simulink library "SingleDotFinder_ul"  (R2018b)
settings: Solver=VariableStepAuto  StartTime=0.0  StopTime=10.0  RelTol=1e-3
undefined symbols (not defined in the file or in its folder): Ignore, masks, vision
libraries: $bdroot x3, simulink x2
settings Model: Creator=mcobb  LastModifiedBy=Owner
settings DebuggingCC: LibraryContextMissingDiagnostic=none
settings SFSimCC: SimUseLocalCustomCode=off
settings RTWCC: RTWUseLocalCustomCode=off

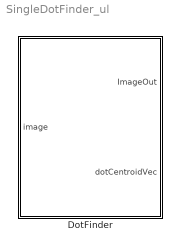
== system SingleDotFinder_ul ==
  DotFinder : Subsystem  mask{ROIPositionHoldEnable=on, ROIPositionHoldCoordinates=[500 500], ROIDimVec_px=[30 90], ROIHalfDimVec_px=[15 45], ROISplitDims_px=[1 15 ; 1 90 ; 16 14 ; 1 90], DotOrientation=Vertical, OverlayOutput=on, ImageDimensions=[765 998], CrosshairPixelWidth_px=1}
      mask prompts: ROIPositionHoldEnable "Hold Position Enable"; ROIPositionHoldCoordinates "Hold Position Coordinates  [rows cols]  (pixels)"; ROIDimVec_px "Dimensions [rows cols]  (pixels)"; ROIHalfDimVec_px "Half Dims  [rows cols]  (pixels)"; ROISplitDims_px "Split Dims [rows cols]  (pixels)"; DotOrientation "Dot Orientation"; OverlayOutput "Draw Output Overlay"; ImageDimensions "Image Dimensions [rows cols] pixels"; CrosshairPixelWidth_px "Crosshair Width (pixels)"
      mask init:
      | dotFinder_init
      mask TypeOptions DotOrientation: Horizontal | Vertical
      mask DialogControl ParameterGroupVar Prompt: Region Of Interest (ROI) Parameters
      mask DialogControl Container3 Prompt: Other Parameters

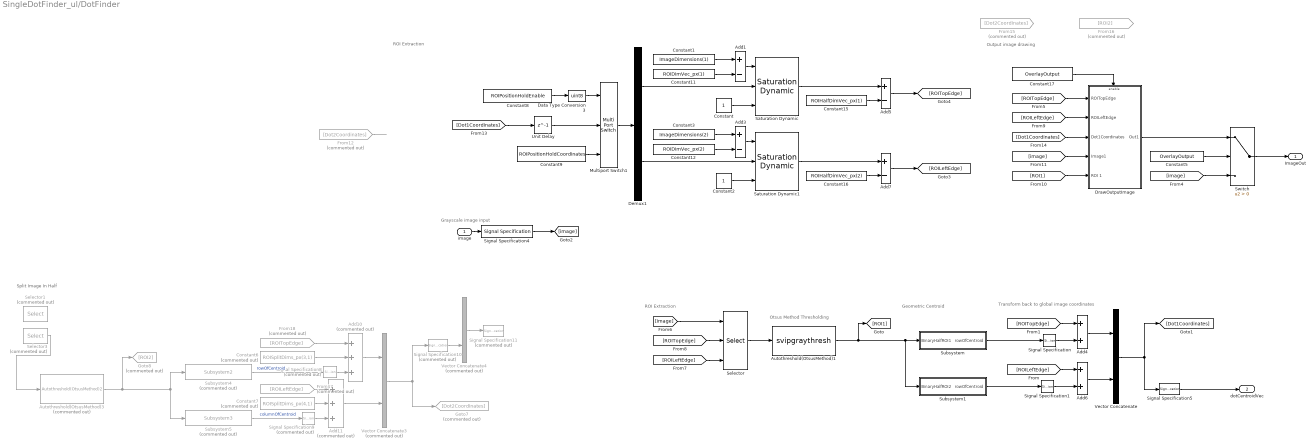
== system SingleDotFinder_ul/DotFinder ==
  note: Transform back to global image coordinates
  note: Geometric Centroid
  note: Otsus Method Thresholding
  note: Split Image
      | In Half
  note: ROI Extraction
  note: Output image drawing
  note: ROI Extraction
  note: Grayscale image input
  image : Inport
  Add{1,3,5,7} (4 alike) : Sum  Inputs=+-
  Add10 : Sum  Commented=on  Inputs=+++
  Add11 : Sum  Commented=on  Inputs=+++
  Add4 : Sum
  Add6 : Sum
  Autothreshold(OtsusMethod)1 : S-Function  DialogController=vipDDGCreate  FunctionName=svipgraythresh  Parameters=operator, userDefinedRange, umin, umax, threshOut, effMetricOut, outOfRngOpt, scaleThreshold, scaleFactor, P1Mode, P1WordLength, P1FracLength, A1Mode, A1WordLength, A1FracLength, P2Mode, P2WordLength, P2FracLength, A2Mode, A2WordLength, A2FracLength, P3Mode, P3WordLength, P3FracLength, A3Mode, A3WordLength, A3FracLength, P4Mode, P4WordLength, P4FracLength, A4Mode, A4WordLength, A4FracLength, Q1Mode, Q1WordLength, Q1FracLength, EMMode, EMWordLength, EMFracLength, dtInfo.roundingMode, dtInfo.overflowMode  SFunctionDeploymentMode=off  EnableBusSupport=off  mask(Autothreshold){operator=>, threshOut=off, effMetricOut=off, userDefinedRange=off, umin=0, umax=255, outOfRngOpt=vision:masks:Ignore, scaleThreshold=off, scaleFactor=1, P1Mode=Specify word length, P1WordLength=32, P1FracLength=30, A1Mode=Same as Product 1, A1WordLength=32, A1FracLength=30, P2Mode=Specify word length, P2WordLength=32, P2FracLength=22, A2Mode=Same as Product 2, A2WordLength=32, A2FracLength=22, P3Mode=Specify word length, P3WordLength=32, P3FracLength=14, A3Mode=Same as Product 3, A3WordLength=32, A3FracLength=14, P4Mode=Binary point scaling, P4WordLength=32, P4FracLength=15, A4Mode=Same as Product 4, A4WordLength=16, A4FracLength=4, Q1Mode=Specify word length, Q1WordLength=32, Q1FracLength=16, EMMode=Specify word length, EMWordLength=16, EMFracLength=14, roundingMode=Floor, overflowMode=off, LockScale=off}
      mask prompts: operator "vision:masks:ThresholdingOperator"; threshOut "vision:masks:OutputThreshold"; effMetricOut "vision:masks:OutputEffectivenessMetric"; userDefinedRange "vision:masks:SpecifyDataRange"; umin "vision:masks:MinimumValueOfInput"; umax "vision:masks:MinimumValueOfInput"; outOfRngOpt "vision:masks:WhenDataRangeIsExceeded"; scaleThreshold "vision:masks:ScaleThreshold_MP"; scaleFactor "vision:masks:ThresholdScalingFactor"; P1Mode "P1:"; P1WordLength "P1 WL:"; P1FracLength "P1 FL:"; A1Mode "A1:"; A1WordLength "A1 WL:"; A1FracLength "A1 FL:"; P2Mode "P2:"; P2WordLength "P2 WL:"; P2FracLength "P2 FL:"; A2Mode "A2:"; A2WordLength "A2 WL:"; A2FracLength "A2 FL:"; P3Mode "P3:"; P3WordLength "P3 WL:"; P3FracLength "P3 FL:"; A3Mode "A3:"; A3WordLength "A3 WL:"; A3FracLength "A3 FL:"; P4Mode "P4:"; P4WordLength "P4 WL:"; P4FracLength "P4 FL:"; A4Mode "A4:"; A4WordLength "A4 WL:"; A4FracLength "A4 FL:"; Q1Mode "Q1:"; Q1WordLength "Q1 WL:"; Q1FracLength "Q1 FL:"; EMMode "EM:"; EMWordLength "EM WL:"; EMFracLength "EM FL:"; roundingMode "vision:masks:RoundIntegerCalculationsTowards"; overflowMode "vision:masks:RoundIntegerCalculationsTowards"; LockScale "vision:masks:LockScaling"
      mask help: vision:masks:AutoThresholdDescription
      mask init:
      | blk = gcbh;
      | 
      | dtInfo = dspGetFixptDataTypeInfo(blk,1);
      | 
      | effMetricOut_str = get_param(blk,'effMetricOut');
      | threshOut_str = get_param(blk,'threshOut');
      | if strcmp(effMetricOut_str,'off') && strcmp(threshOut_str,'off')
      | 	[so(1:3).port] = deal(1,1,1);
      | 	[so(1:3).txt] = deal('BW','BW','BW');
      | elseif strcmp(effMetricOut_str,'on') && strcmp(threshOut_str,'off')
      | 	[so(1:3).port] = deal(1,2,2);
      | 	[so(1:3).txt] = deal('BW','EMetric','EMetric');
      | elseif strcmp(effMetricOut_str,'off') && strcmp(threshOut_str,'on')
      | 	[so(1:3).port] = deal(1,2,2);
      | 	[so(1:3).txt] = deal('BW','Th','Th');
      | else
      | 	[so(1:3).port] = deal(1,2,3);
      | 	[so(1:3).txt] = deal('BW','Th','EMetric');
      | end
      mask Help: eval('visionblockhelp');
      mask TypeOptions operator: > | <=
      mask TypeOptions outOfRngOpt: vision:masks:Ignore | vision:masks:Saturate | vision:masks:WarnAndSaturate | vision:masks:Error
      mask TypeOptions P1Mode: Specify word length | Binary point scaling | Slope and bias scaling
      mask TypeOptions A1Mode: Same as Product 1 | Specify word length | Binary point scaling | Slope and bias scaling
      mask TypeOptions P2Mode: Specify word length | Binary point scaling | Slope and bias scaling
      mask TypeOptions A2Mode: Same as Product 2 | Specify word length | Binary point scaling | Slope and bias scaling
      mask TypeOptions P3Mode: Specify word length | Binary point scaling | Slope and bias scaling
      mask TypeOptions A3Mode: Same as Product 3 | Specify word length | Binary point scaling | Slope and bias scaling
      mask TypeOptions P4Mode: Same as input | Binary point scaling | Slope and bias scaling
      mask TypeOptions A4Mode: Same as Product 4 | Binary point scaling | Slope and bias scaling
      mask TypeOptions Q1Mode: Specify word length | Binary point scaling | Slope and bias scaling
      mask TypeOptions EMMode: Specify word length | Binary point scaling | Slope and bias scaling
      mask TypeOptions roundingMode: dspshared:FixptDialog:Ceiling_CB | dspshared:FixptDialog:Convergent_CB | dspshared:FixptDialog:Floor_CB | dspshared:FixptDialog:Nearest_CB | dspshared:FixptDialog:Round_CB | dspshared:FixptDialog:Simplest_CB | dspshared:FixptDialog:Zero_CB
      mask Display:
      | disp('Autothreshold');
      | port_label('input',1,'I');
      | port_label('output',so(1).port, so(1).txt);
      | port_label('output',so(2).port, so(2).txt);
      | port_label('output',so(3).port, so(3).txt);
  Autothreshold(OtsusMethod)3 : $bdroot/DotFinder/Autothreshold(OtsusMethod)2  Commented=on  operator=>  threshOut=off  effMetricOut=off  userDefinedRange=off  umin=0  umax=255  outOfRngOpt=vision:masks:Ignore  scaleThreshold=off  scaleFactor=1  P1Mode=Specify word length  P1WordLength=32  P1FracLength=30  P2Mode=Specify word length  P2WordLength=32  P2FracLength=22  P3Mode=Specify word length  P3WordLength=32  P3FracLength=14  P4Mode=Binary point scaling  P4WordLength=32  P4FracLength=15  Q1Mode=Specify word length  Q1WordLength=32  Q1FracLength=16  EMMode=Specify word length  EMWordLength=16  EMFracLength=14  roundingMode=Floor  overflowMode=off
  Constant : Constant
  Constant1 : Constant  Value=ImageDimensions(1)
  Constant11 : Constant  Value=ROIDimVec_px(1)
  Constant12 : Constant  Value=ROIDimVec_px(2)
  Constant15 : Constant  Value=ROIHalfDimVec_px(1)
  Constant16 : Constant  Value=ROIHalfDimVec_px(2)
  Constant17 : Constant  Value=OverlayOutput
  Constant2 : Constant
  Constant3 : Constant  Value=ImageDimensions(2)
  Constant5 : Constant  Value=OverlayOutput
  Constant6 : Constant  Commented=on  Value=ROISplitDims_px(3,1)
  Constant7 : Constant  Commented=on  Value=ROISplitDims_px(4,1)
  Constant8 : Constant  Value=ROIPositionHoldEnable
  Constant9 : Constant  Value=ROIPositionHoldCoordinates
  Data Type Conversion3 : DataTypeConversion  OutDataTypeStr=uint8
  Demux1 : Demux  Outputs=2
  DrawOutputImage : Subsystem
  From12 : From  Commented=on  GotoTag=Dot2Coordinates
  From15 : From  Commented=on  GotoTag=Dot2Coordinates
  From16 : From  Commented=on  GotoTag=ROI2
  From17 : From  Commented=on  GotoTag=ROILeftEdge
  From18 : From  Commented=on  GotoTag=ROITopEdge
  Goto7 : Goto  Commented=on  GotoTag=Dot2Coordinates
  Goto8 : Goto  Commented=on  GotoTag=ROI2
  Multiport Switch1 : MultiPortSwitch  DataPortOrder=Zero-based contiguous  Inputs=2  zeroidx=on
  Saturation Dynamic : simulink/Discontinuities/Saturation Dynamic  OutMin=[]  OutMax=[]  OutDataTypeStr=Inherit: Same as second input  OutDataType=fixdt(1, 16)  OutScaling=2^-10  DoSatur=off
  Saturation Dynamic1 : simulink/Discontinuities/Saturation Dynamic  OutMin=[]  OutMax=[]  OutDataTypeStr=Inherit: Same as second input  OutDataType=fixdt(1, 16)  OutScaling=2^-10  DoSatur=off
  Selector : Selector  NumberOfDimensions=2  InputPortWidth=3  IndexOptions=Starting index (port),Starting index (port)  Indices=[1 3],1  OutputSizes=ROIDimVec_px(1),ROIDimVec_px(2)
  Selector1 : Selector  Commented=on  NumberOfDimensions=2  InputPortWidth=3  IndexOptions=Starting index (dialog),Starting index (dialog)  Indices=ROISplitDims_px(1,1),ROISplitDims_px(2,1)  OutputSizes=ROISplitDims_px(1,2),ROISplitDims_px(2,2)
  Selector3 : Selector  Commented=on  NumberOfDimensions=2  InputPortWidth=3  IndexOptions=Starting index (dialog),Starting index (dialog)  Indices=ROISplitDims_px(3,1),ROISplitDims_px(4,1)  OutputSizes=ROISplitDims_px(3,2),ROISplitDims_px(4,2)
  Signal Specification : SignalSpecification  Dimensions=1
  Signal Specification1 : SignalSpecification  Dimensions=1
  Signal Specification10 : SignalSpecification  Commented=on  Dimensions=[1 2]
  Signal Specification11 : SignalSpecification  Commented=on  Dimensions=[1 4]
  Signal Specification4 : SignalSpecification  Dimensions=ImageDimensions
  Signal Specification5 : SignalSpecification  Dimensions=[1 2]
  Signal Specification8 : SignalSpecification  Commented=on  Dimensions=1
  Signal Specification9 : SignalSpecification  Commented=on  Dimensions=1
  Subsystem : Subsystem
  Subsystem1 : Subsystem
  Subsystem4 : $bdroot/DotFinder/Subsystem2  Commented=on  SystemSampleTime=-1  SSRTWFcnClass=[]
  Subsystem5 : $bdroot/DotFinder/Subsystem3  Commented=on  SystemSampleTime=-1  SSRTWFcnClass=[]
  Switch : Switch  Criteria=u2 > Threshold
  Unit Delay : Delay  DelayLength=1  InitialCondition=ROIPositionHoldCoordinates
  Vector Concatenate : Concatenate
  Vector Concatenate3 : Concatenate  Commented=on
  Vector Concatenate4 : Concatenate  Commented=on  ConcatenateDimension=2
  ImageOut : Outport  PortDimensions=ImageDimensions
  dotCentroidVec : Outport  Port=2
  wires:
  Data Type Conversion3/1 -> Multiport Switch1/1
  Unit Delay/1 -> Multiport Switch1/2
  Multiport Switch1/1 -> Demux1/1
  Demux1/1 -> Saturation Dynamic/2
  Constant/1 -> Saturation Dynamic/3
  Constant1/1 -> Add1/1
  Constant11/1 -> Add1/2
  Constant12/1 -> Add3/2
  Constant3/1 -> Add3/1
  Demux1/2 -> Saturation Dynamic1/2
  Constant15/1 -> Add5/2
  Constant16/1 -> Add7/2
  [image] -> Selector/1
  Constant8/1 -> Data Type Conversion3/1
  Constant9/1 -> Multiport Switch1/3
  Saturation Dynamic/1 -> Add5/1
  Saturation Dynamic1/1 -> Add7/1
  Constant2/1 -> Saturation Dynamic1/3
  Add3/1 -> Saturation Dynamic1/1
  Add1/1 -> Saturation Dynamic/1
  Subsystem1/1(rowOfCentroid) -> Signal Specification1/1
  [ROITopEdge] -> Add4/1
  [ROILeftEdge] -> Add6/1
  Add4/1 -> Vector Concatenate/1
  Add6/1 -> Vector Concatenate/2
  image/1 -> Signal Specification4/1
  Add7/1 -> [ROILeftEdge]
  Add5/1 -> [ROITopEdge]
  Constant17/1 -> DrawOutputImage/Enable
  DrawOutputImage/1(Out1) -> Switch/1
  [ROILeftEdge] -> Selector/3
  [ROITopEdge] -> Selector/2
  [ROITopEdge] -> DrawOutputImage/1(ROITopEdge)
  [ROILeftEdge] -> DrawOutputImage/2(ROILeftEdge)
  [ROI1] -> DrawOutputImage/5("ROI 1 ")
  [image] -> Switch/3
  Constant5/1 -> Switch/2
  [image] -> DrawOutputImage/4(Image1)
  Vector Concatenate/1 -> Signal Specification5/1, [Dot1Coordinates]
  [Dot1Coordinates] -> DrawOutputImage/3(Dot1Coordinates)
  Switch/1 -> ImageOut/1
  Signal Specification/1 -> Add4/2
  Signal Specification1/1 -> Add6/2
  Signal Specification4/1 -> [image]
  Subsystem/1(rowOfCentroid) -> Signal Specification/1
  Autothreshold(OtsusMethod)1/1 -> [ROI1], Subsystem1/1(BinaryHalfROI2), Subsystem/1(BinaryHalfROI1)
  From12/1 -> ?
  [Dot1Coordinates] -> Unit Delay/1
  Signal Specification10/1 -> Vector Concatenate4/2
  Vector Concatenate4/1 -> Signal Specification11/1
  Autothreshold(OtsusMethod)3/1 -> Subsystem4/1, Subsystem5/1, Goto8/1
  Signal Specification9/1 -> Add11/3
  Signal Specification8/1 -> Add10/3
  Vector Concatenate3/1 -> Goto7/1, Signal Specification10/1
  Constant6/1 -> Add10/2
  Constant7/1 -> Add11/2
  Selector3/1 -> Autothreshold(OtsusMethod)3/1
  Subsystem4/1 -> Signal Specification8/1  "rowOfCentroid"
  Subsystem5/1 -> Signal Specification9/1  "columnOfCentroid"
  From18/1 -> Add10/1
  From17/1 -> Add11/1
  Add10/1 -> Vector Concatenate3/1
  Add11/1 -> Vector Concatenate3/2
  Signal Specification5/1 -> dotCentroidVec/1
  Selector/1 -> Autothreshold(OtsusMethod)1/1

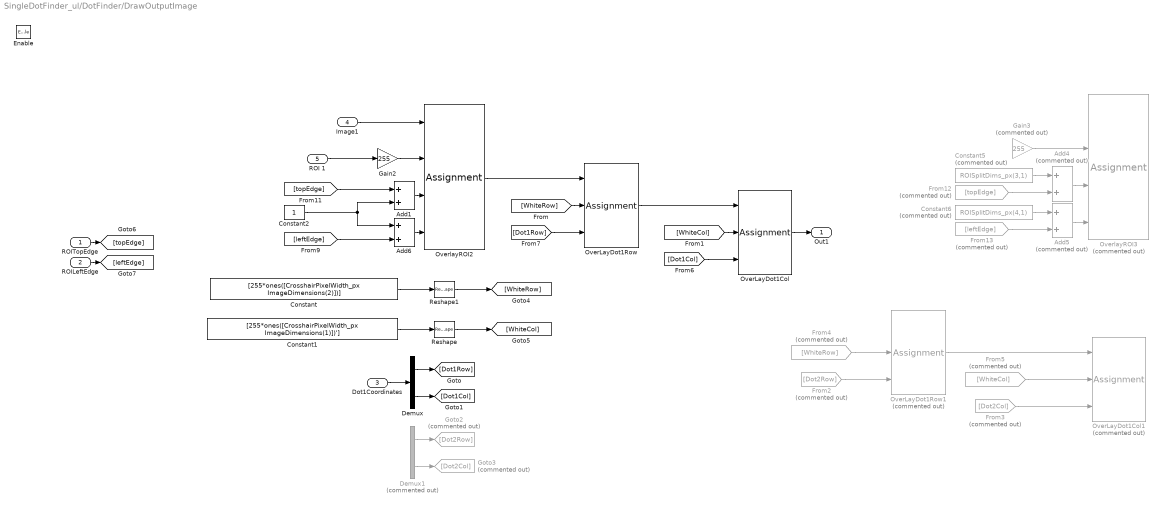
== system SingleDotFinder_ul/DotFinder/DrawOutputImage ==
  ROITopEdge : Inport
  ROILeftEdge : Inport  Port=2
  Dot1Coordinates : Inport  Port=3  PortDimensions=2
  Image1 : Inport  Port=4
  "ROI 1 " : Inport  Port=5
  Enable : EnablePort
  Add1 : Sum
  Add4 : Sum  Commented=on
  Add5 : Sum  Commented=on
  Add6 : Sum
  Constant : Constant  Value=[255*ones([CrosshairPixelWidth_px ImageDimensions(2)])]  OutDataTypeStr=uint8
  Constant1 : Constant  Value=[255*ones([CrosshairPixelWidth_px ImageDimensions(1)])']  OutDataTypeStr=uint8
  Constant2 : Constant
  Constant5 : Constant  Commented=on  Value=ROISplitDims_px(3,1)
  Constant6 : Constant  Commented=on  Value=ROISplitDims_px(4,1)
  Demux : Demux  Outputs=2
  Demux1 : Demux  Commented=on  Outputs=2
  From12 : From  Commented=on  GotoTag=topEdge
  From13 : From  Commented=on  GotoTag=leftEdge
  From2 : From  Commented=on  GotoTag=Dot2Row
  From3 : From  Commented=on  GotoTag=Dot2Col
  From4 : From  Commented=on  GotoTag=WhiteRow
  From5 : From  Commented=on  GotoTag=WhiteCol
  Gain2 : Gain  Gain=255  OutDataTypeStr=uint8
  Gain3 : Gain  Commented=on  Gain=255  OutDataTypeStr=uint8
  Goto2 : Goto  Commented=on  GotoTag=Dot2Row
  Goto3 : Goto  Commented=on  GotoTag=Dot2Col
  OverLayDot1Col : Assignment  NumberOfDimensions=2  DiagnosticForDimensions=Warning  IndexOptions=Assign all,Starting index (port)  Indices=1,1  OutputSizes=1,1
  OverLayDot1Col1 : Assignment  Commented=on  NumberOfDimensions=2  DiagnosticForDimensions=Warning  IndexOptions=Assign all,Starting index (port)  Indices=1,1  OutputSizes=1,1
  OverLayDot1Row : Assignment  NumberOfDimensions=2  DiagnosticForDimensions=Warning  IndexOptions=Starting index (port),Assign all  Indices=1,1  OutputSizes=1,1
  OverLayDot1Row1 : Assignment  Commented=on  NumberOfDimensions=2  DiagnosticForDimensions=Warning  IndexOptions=Starting index (port),Assign all  Indices=1,1  OutputSizes=1,1
  OverlayROI2 : Assignment  NumberOfDimensions=2  DiagnosticForDimensions=Warning  IndexOptions=Starting index (port),Starting index (port)  Indices=1,1  OutputSizes=1,1
  OverlayROI3 : Assignment  Commented=on  NumberOfDimensions=2  DiagnosticForDimensions=Warning  IndexOptions=Starting index (port),Starting index (port)  Indices=1,1  OutputSizes=1,1
  Reshape : Reshape  OutputDimensionality=Customize  OutputDimensions=[ImageDimensions(1) CrosshairPixelWidth_px ]
  Reshape1 : Reshape  OutputDimensionality=Customize  OutputDimensions=[CrosshairPixelWidth_px ImageDimensions(2)]
  Out1 : Outport
  wires:
  Dot1Coordinates/1 -> Demux/1
  Demux/1 -> [Dot1Row]
  Demux/2 -> [Dot1Col]
  Demux1/1 -> Goto2/1
  Demux1/2 -> Goto3/1
  Constant/1 -> Reshape1/1
  Constant1/1 -> Reshape/1
  OverLayDot1Row/1 -> OverLayDot1Col/1
  OverLayDot1Row1/1 -> OverLayDot1Col1/1
  [WhiteRow] -> OverLayDot1Row/2
  [WhiteCol] -> OverLayDot1Col/2
  From2/1 -> OverLayDot1Row1/3
  From3/1 -> OverLayDot1Col1/3
  From4/1 -> OverLayDot1Row1/2
  From5/1 -> OverLayDot1Col1/2
  [Dot1Col] -> OverLayDot1Col/3
  [Dot1Row] -> OverLayDot1Row/3
  Reshape1/1 -> [WhiteRow]
  Reshape/1 -> [WhiteCol]
  ROITopEdge/1 -> [topEdge]
  ROILeftEdge/1 -> [leftEdge]
  OverLayDot1Col/1 -> Out1/1
  From12/1 -> Add4/2
  From13/1 -> Add5/2
  Constant6/1 -> Add5/1
  Constant5/1 -> Add4/1
  Add5/1 -> OverlayROI3/4
  Add4/1 -> OverlayROI3/3
  Gain3/1 -> OverlayROI3/2
  "ROI 1 "/1 -> Gain2/1
  Constant2/1 -> Add1/2, Add6/1
  [leftEdge] -> Add6/2
  [topEdge] -> Add1/1
  Add6/1 -> OverlayROI2/4
  Add1/1 -> OverlayROI2/3
  Image1/1 -> OverlayROI2/1
  Gain2/1 -> OverlayROI2/2
  OverlayROI2/1 -> OverLayDot1Row/1

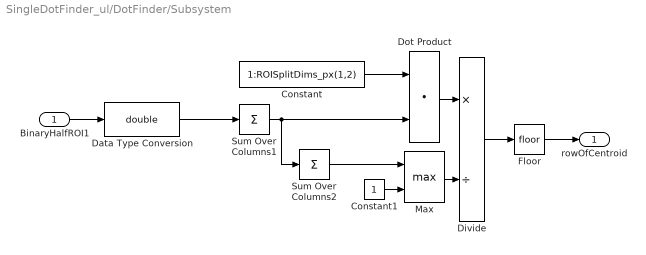
== system SingleDotFinder_ul/DotFinder/Subsystem ==
  BinaryHalfROI1 : Inport
  Constant : Constant  Value=1:ROISplitDims_px(1,2)
  Constant1 : Constant
  Data Type Conversion : DataTypeConversion  OutDataTypeStr=double
  Divide : Product  Inputs=*/
  Dot Product : DotProduct  InputSameDT=on  OutDataTypeStr=Inherit: Inherit via internal rule
  Floor : Rounding
  Max : MinMax  Function=max  Inputs=2
  Sum Over Columns1 : Sum  Inputs=+  CollapseMode=Specified dimension  CollapseDim=2
  Sum Over Columns2 : Sum  Inputs=+  CollapseDim=2
  rowOfCentroid : Outport
  wires:
  BinaryHalfROI1/1 -> Data Type Conversion/1
  Divide/1 -> Floor/1
  Constant/1 -> Dot Product/1
  Dot Product/1 -> Divide/1
  Sum Over Columns1/1 -> Sum Over Columns2/1, Dot Product/2
  Sum Over Columns2/1 -> Max/1
  Max/1 -> Divide/2
  Constant1/1 -> Max/2
  Floor/1 -> rowOfCentroid/1
  Data Type Conversion/1 -> Sum Over Columns1/1

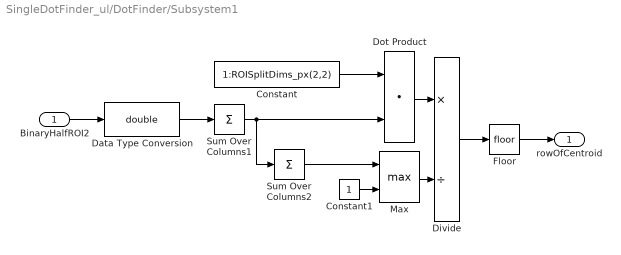
== system SingleDotFinder_ul/DotFinder/Subsystem1 ==
  BinaryHalfROI2 : Inport
  Constant : Constant  Value=1:ROISplitDims_px(2,2)
  Constant1 : Constant
  Data Type Conversion : DataTypeConversion  OutDataTypeStr=double
  Divide : Product  Inputs=*/
  Dot Product : DotProduct  InputSameDT=on  OutDataTypeStr=Inherit: Inherit via internal rule
  Floor : Rounding
  Max : MinMax  Function=max  Inputs=2
  Sum Over Columns1 : Sum  Inputs=+  CollapseMode=Specified dimension
  Sum Over Columns2 : Sum  Inputs=+  CollapseDim=2
  rowOfCentroid : Outport
  wires:
  Floor/1 -> rowOfCentroid/1
  Constant1/1 -> Max/2
  Max/1 -> Divide/2
  Sum Over Columns2/1 -> Max/1
  Sum Over Columns1/1 -> Dot Product/2, Sum Over Columns2/1
  Dot Product/1 -> Divide/1
  Constant/1 -> Dot Product/1
  Divide/1 -> Floor/1
  BinaryHalfROI2/1 -> Data Type Conversion/1
  Data Type Conversion/1 -> Sum Over Columns1/1
